simulink model "CA3"  (R2024b)
settings: Solver=VariableStepAuto  StartTime=0.0  StopTime=120.0  RelTol=1e-3
values from neighbouring files (symbols this model uses):
  b = [0;1]    [Parameters.m]
  C = 0.7    [Parameters.m]
  Gamma = [1 0;0 1]    [Parameters.m]
  gamma = 1    [Parameters.m]
  K = 6.2    [Parameters.m]
  noise_gain_x1 = 0.0    (= 0)    [Parameters.m]
  noise_gain_x2 = 0.0    (= 0)    [Parameters.m]
  P = lyap(Am', Q)    [Parameters.m]    (also in calibration.m = (theta_rad'*theta_rad)^(-1))
  tau = 0.25    [Parameters.m]
  w = 5    [Parameters.m]
settings Model: Creator=xym  LastModifiedBy=xym

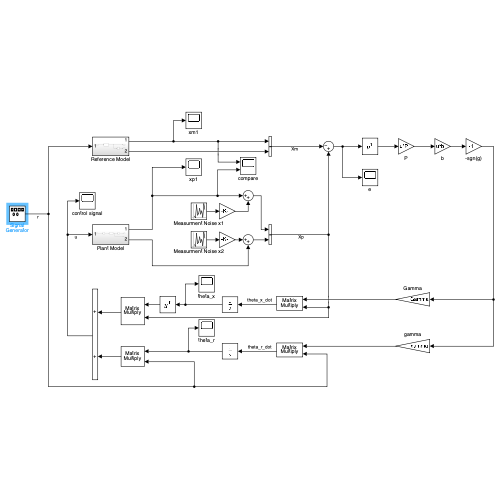
[thumbnail: Simulink's stored preview of the top-level diagram]
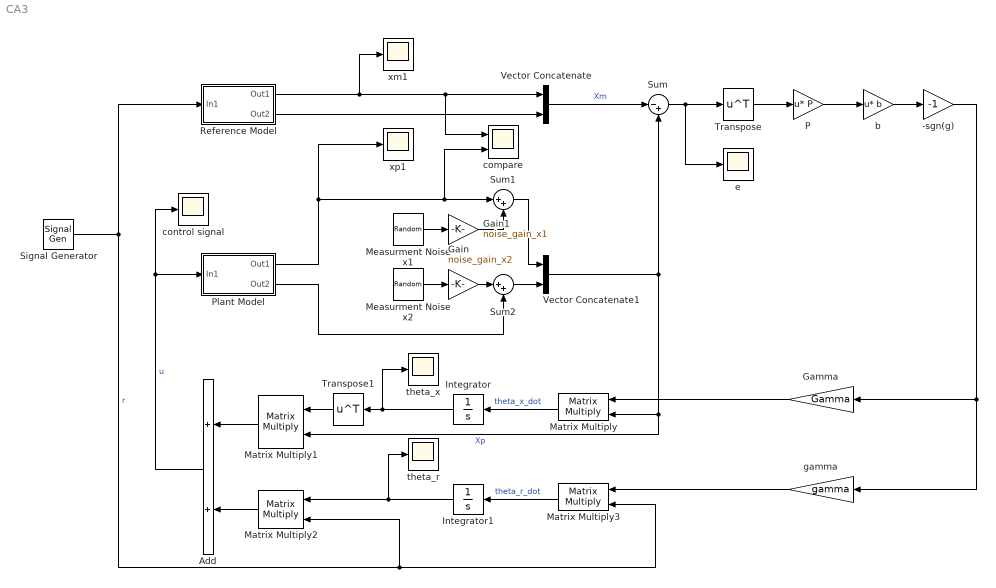
== system CA3 ==
  -sgn(g) : Gain  Gain=-1
  Add : Sum
  Gain : Gain  Gain=noise_gain_x2
  Gain1 : Gain  Gain=noise_gain_x1
  Gamma : Gain  Gain=Gamma
  Integrator : Integrator
  Integrator1 : Integrator
  Matrix Multiply{,1..3} (4 alike) : Product  Multiplication=Matrix(*)
  Measurment Noise x1 : UniformRandomNumber  SampleTime=0.1
  Measurment Noise x2 : UniformRandomNumber  SampleTime=0.1
  P : Gain  Gain=P  Multiplication=Matrix(u*K)
  Plant Model : Subsystem
  Reference Model : Subsystem
  Signal Generator : SignalGenerator  Frequency=0.5  Units=rad/sec
  Sum : Sum  Inputs=|-+
  Sum1 : Sum  Inputs=|++
  Sum2 : Sum  Inputs=|++
  Transpose : Math  Operator=transpose
  Transpose1 : Math  Operator=transpose
  Vector Concatenate : Concatenate
  Vector Concatenate1 : Concatenate
  b : Gain  Gain=b  Multiplication=Matrix(u*K)
  compare : Scope  NumInputPorts=2
  control signal : Scope
  e : Scope
  gamma : Gain  Gain=gamma
  theta_r : Scope
  theta_x : Scope
  xm1 : Scope
  xp1 : Scope
  wires:
  Signal Generator/1 -> Matrix Multiply2/2, Matrix Multiply3/2, Reference Model/1(In1)  "r"
  Reference Model/1(Out1) -> Vector Concatenate/1, compare/1, xm1/1
  Reference Model/2(Out2) -> Vector Concatenate/2
  Vector Concatenate/1 -> Sum/1  "Xm"
  Sum/1 -> Transpose/1, e/1
  Transpose/1 -> P/1
  P/1 -> b/1
  b/1 -> -sgn(g)/1
  Plant Model/2(Out2) -> Sum2/2
  Vector Concatenate1/1 -> Matrix Multiply1/2, Matrix Multiply/2, Sum/2  "Xp"
  -sgn(g)/1 -> gamma/1, Gamma/1
  Gamma/1 -> Matrix Multiply/1
  Matrix Multiply/1 -> Integrator/1  "theta_x_dot"
  Integrator/1 -> theta_x/1, Transpose1/1
  Transpose1/1 -> Matrix Multiply1/1
  Matrix Multiply1/1 -> Add/1
  Matrix Multiply2/1 -> Add/2
  gamma/1 -> Matrix Multiply3/1
  Matrix Multiply3/1 -> Integrator1/1  "theta_r_dot"
  Integrator1/1 -> theta_r/1, Matrix Multiply2/1
  Plant Model/1(Out1) -> compare/2, Sum1/1, xp1/1
  Sum1/1 -> Vector Concatenate1/1
  Sum2/1 -> Vector Concatenate1/2
  Measurment Noise x2/1 -> Gain/1
  Measurment Noise x1/1 -> Gain1/1
  Gain1/1 -> Sum1/2
  Gain/1 -> Sum2/1
  Add/1 -> Plant Model/1(In1), control signal/1  "u"

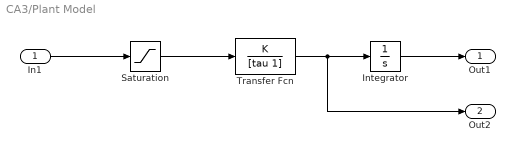
== system CA3/Plant Model ==
  In1 : Inport
  Integrator : Integrator
  Saturation : Saturate  UpperLimit=5  LowerLimit=-5
  Transfer Fcn : TransferFcn  Numerator=K  Denominator=[tau 1]
  Out1 : Outport
  Out2 : Outport  Port=2
  wires:
  Integrator/1 -> Out1/1
  Saturation/1 -> Transfer Fcn/1
  In1/1 -> Saturation/1
  Transfer Fcn/1 -> Out2/1, Integrator/1

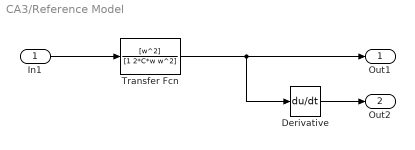
== system CA3/Reference Model ==
  In1 : Inport
  Derivative : Derivative
  Transfer Fcn : TransferFcn  Numerator=[w^2]  Denominator=[1 2*C*w w^2]
  Out1 : Outport
  Out2 : Outport  Port=2
  wires:
  In1/1 -> Transfer Fcn/1
  Transfer Fcn/1 -> Out1/1, Derivative/1
  Derivative/1 -> Out2/1
